simulink library "tether005_ul"  (R2020a)
settings: Solver=VariableStepAuto  StartTime=0.0  StopTime=10.0  RelTol=1e-3
values from neighbouring files (symbols this model uses):
  initNodePos = [INITIALLINE;INITIALLINE;INITIALLINE]    [tether005_ts.m]
  initNodeVel = [zeros(1,numNodes-2);zeros(1,numNodes-2);zeros(1,numNodes-2)]    [tether005_ts.m]
  numNodes = 11    [tether005_ts.m]
libraries: powerlib_meascontrol x2
settings Model: Creator=mitch  LastModifiedBy=mr-jo

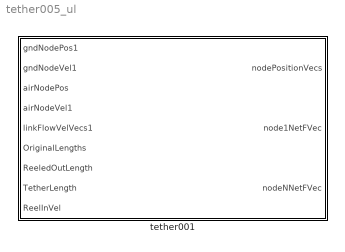
== system tether005_ul ==
  tether001 : Subsystem

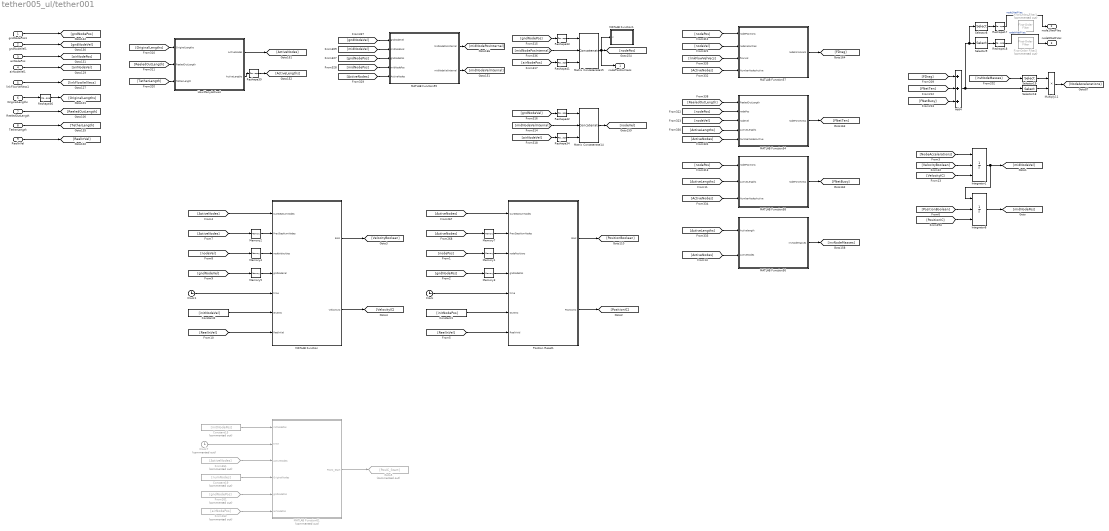
== system tether005_ul/tether001 ==
  gndNodePos1 : Inport
  gndNodeVel1 : Inport  Port=2
  airNodePos : Inport  Port=3
  airNodeVel1 : Inport  Port=4
  linkFlowVelVecs1 : Inport  Port=5
  OriginalLengths : Inport  Port=6
  ReeledOutLength : Inport  Port=7
  TetherLength : Inport  Port=8
  ReelInVel : Inport  Port=9
  Add4 : Sum  Inputs=3
  Clock : Clock
  Clock1 : Clock
  Clock7 : Clock  Commented=on
  Constant1 : Constant  Value=[initNodePos]
  Constant15 : Constant  Commented=on  Value=[initNodePos]
  Constant19 : Constant  Commented=on  Value=[numNodes]
  Constant2 : Constant  Value=[initNodeVel]
  First-Order Filter1 : powerlib_meascontrol/Filters/First-Order Filter  Commented=on  FilterType=Lowpass  Tc=1  Ts=0  Initialize=on  Vac_Init=[0, 0, 60]  Vdc_Init=0  PlotResponse=off  FreqRange="[0,  200,  1]"
  First-Order Filter2 : powerlib_meascontrol/Filters/First-Order Filter  Commented=on  FilterType=Lowpass  Tc=1  Ts=0  Initialize=on  Vac_Init=[0, 0, 60]  Vdc_Init=0  PlotResponse=off  FreqRange="[0,  200,  1]"
  From161 : From  Commented=on  GotoTag=gndNodePos
  From162 : From  Commented=on  GotoTag=airNodePos
  From361 : From  Commented=on  GotoTag=ActiveNodes
  Goto5 : Goto  Commented=on  GotoTag=PosIC_Start
  HowManyActive4 : MATLAB Function  TreatAsAtomicUnit=on
  Integrator1 : Integrator  ExternalReset=rising  InitialConditionSource=external
  Integrator8 : Integrator  ExternalReset=rising  InitialConditionSource=external
  MATLAB Function : MATLAB Function  TreatAsAtomicUnit=on
  MATLAB Function1 : MATLAB Function  TreatAsAtomicUnit=on
  MATLAB Function54 : MATLAB Function  TreatAsAtomicUnit=on
  MATLAB Function55 : MATLAB Function  TreatAsAtomicUnit=on
  MATLAB Function56 : MATLAB Function  TreatAsAtomicUnit=on
  MATLAB Function57 : MATLAB Function  TreatAsAtomicUnit=on
  MATLAB Function58 : MATLAB Function  TreatAsAtomicUnit=on
  MATLAB Function61 : MATLAB Function  Commented=on  TreatAsAtomicUnit=on
  Matrix Concatenate14 : Concatenate  NumInputs=3  Mode=Multidimensional array  ConcatenateDimension=2
  Matrix Concatenate15 : Concatenate  NumInputs=3  Mode=Multidimensional array  ConcatenateDimension=2
  Memory{1..5,7} (6 alike) : Memory
  Multiply11 : Product
  Position Reset1 : MATLAB Function  TreatAsAtomicUnit=on
  Reshape{17..18,33..34,41..42} (6 alike) : Reshape  OutputDimensionality=Column vector (2-D)
  Reshape36 : Reshape  OutputDimensionality=Row vector (2-D)
  Reshape39 : Reshape  OutputDimensionality=Row vector (2-D)
  Selector18 : Selector  NumberOfDimensions=2  InputPortWidth=3  IndexOptions=Select all,Index vector (dialog)  Indices=[1 3],2:numNodes-1  OutputSizes=1,1
  Selector19 : Selector  NumberOfDimensions=2  InputPortWidth=3  IndexOptions=Select all,Index vector (dialog)  Indices=[1 3],2:numNodes-1  OutputSizes=1,1
  Selector8 : Selector  NumberOfDimensions=2  InputPortWidth=3  IndexOptions=Select all,Index vector (dialog)  Indices=[1 3],1  OutputSizes=1,1
  Selector9 : Selector  NumberOfDimensions=2  InputPortWidth=3  IndexOptions=Select all,Starting index (dialog)  Indices=[1 3],numNodes  OutputSizes=1,1
  nodePositionVecs : Outport  VectorParamsAs1DForOutWhenUnconnected=off
  node1NetFVec : Outport  Port=2  VectorParamsAs1DForOutWhenUnconnected=off
  nodeNNetFVec : Outport  Port=3  VectorParamsAs1DForOutWhenUnconnected=off
  wires:
  ? -> ?
  [gndNodeVel] -> Reshape42/1
  [ActiveNodes] -> MATLAB Function54/5(NumberNodesActive)
  MATLAB Function56/1(invNodeMasses) -> [invNodeMasses]
  [gndNodePos] -> Reshape33/1
  HowManyActive4/2(ActiveLengths) -> Reshape39/1
  [airNodePos] -> Reshape41/1
  [midNodePosInternal] -> Matrix Concatenate15/2
  [nodePos] -> MATLAB Function57/1(nodePositions)
  [ActiveLengths] -> MATLAB Function56/1(Activelength)
  MATLAB Function58/1(nodeForceVecs) -> [FNetBuoy]
  [ReeledOutLength] -> HowManyActive4/2(ReeledOutLength)
  Reshape42/1 -> Matrix Concatenate14/1
  [ActiveNodes] -> MATLAB Function58/3(NumberNodesActive)
  Reshape39/1 -> [ActiveLengths]
  Reshape41/1 -> Matrix Concatenate15/3
  Reshape33/1 -> Matrix Concatenate15/1
  [airNodeVel] -> Reshape34/1
  [nodeVel] -> MATLAB Function54/3(nodeVel)
  Matrix Concatenate14/1 -> [nodeVel]
  MATLAB Function54/1(nodeForceVecs) -> [FNetTen]
  [nodePos] -> MATLAB Function58/1(nodePositions)
  Matrix Concatenate15/1 -> MATLAB Function1/1(u), [nodePos], nodePositionVecs/1
  [ActiveLengths] -> MATLAB Function54/4(ActiveLengths)
  [gndNodeVel] -> MATLAB Function55/1(gndNodeVel)
  HowManyActive4/1(ActiveNodes) -> [ActiveNodes]
  [midNodePos] -> MATLAB Function55/4(midNodePos)
  [ActiveNodes] -> MATLAB Function55/5(ActiveNodes)
  [midNodeVelInternal] -> Matrix Concatenate14/2
  [gndNodePos] -> MATLAB Function55/3(gndNodePos)
  Reshape34/1 -> Matrix Concatenate14/3
  [nodeVel] -> MATLAB Function57/2(nodeVelocities)
  [TetherLength] -> HowManyActive4/3(TetherLength)
  [ActiveNodes] -> MATLAB Function57/4(NumberNodesActive)
  [ReeledOutLength] -> MATLAB Function54/1(ReeledOutLength)
  MATLAB Function55/2(midNodeVelInternal) -> [midNodeVelInternal]
  [nodePos] -> MATLAB Function54/2(nodePos)
  [midNodeVel] -> MATLAB Function55/2(midNodeVel)
  MATLAB Function57/1(nodeForceVecs) -> [FDrag]
  [linkFlowVelVecs] -> MATLAB Function57/3(flowVel)
  [OriginalLengths] -> HowManyActive4/1(OriginalLengths)
  ReeledOutLength/1 -> [ReeledOutLength]
  Reshape36/1 -> [OriginalLengths]
  gndNodePos1/1 -> [gndNodePos]
  gndNodeVel1/1 -> [gndNodeVel]
  airNodePos/1 -> [airNodePos]
  airNodeVel1/1 -> [airNodeVel]
  linkFlowVelVecs1/1 -> [linkFlowVelVecs]
  OriginalLengths/1 -> Reshape36/1
  TetherLength/1 -> [TetherLength]
  ReelInVel/1 -> [ReelInVel]
  MATLAB Function55/1(midNodePosInternal) -> [midNodePosInternal]
  [ActiveNodes] -> Position Reset1/1(CurStepNumNodes)
  Position Reset1/1(Bool) -> [PositionBoolean]
  [ActiveNodes] -> Memory7/1
  Selector18/1 -> Multiply11/2
  Memory7/1 -> Position Reset1/2(PrevStepNumNodes)
  [invNodeMasses] -> Selector19/1
  Selector19/1 -> Multiply11/1
  [FNetTen] -> Add4/2
  Add4/1 -> Selector9/1, Selector8/1, Selector18/1
  [FDrag] -> Add4/1
  Multiply11/1 -> [NodeAccelerations]
  [FNetBuoy] -> Add4/3
  [NodeAccelerations] -> Integrator1/1
  Integrator8/1 -> [midNodePos]
  [gndNodePos] -> Memory3/1
  Position Reset1/2(PositionIC) -> [PositionIC]
  Clock/1 -> Position Reset1/5(time)
  [PositionIC] -> Integrator8/3
  Memory3/1 -> Position Reset1/4(gndNodePos)
  [ReelInVel] -> Position Reset1/7(ReelInVel)
  Selector8/1 -> Reshape17/1
  Selector9/1 -> Reshape18/1
  Integrator1/1 -> Integrator8/1, [midNodeVel]
  [PositionBoolean] -> Integrator8/2
  [ActiveNodes] -> MATLAB Function/1(CurStepNumNodes)
  [ActiveNodes] -> Memory2/1
  Memory2/1 -> MATLAB Function/2(PrevStepNumNodes)
  [nodeVel] -> Memory4/1
  Memory4/1 -> MATLAB Function/3(nodeVelocities)
  [gndNodeVel] -> Memory5/1
  Memory5/1 -> MATLAB Function/4(gndNodeVel)
  Clock1/1 -> MATLAB Function/5(time)
  Constant2/1 -> MATLAB Function/6(GivenIC)
  [ReelInVel] -> MATLAB Function/7(ReelInVel)
  MATLAB Function/1(Bool) -> [VelocityBoolean]
  MATLAB Function/2(VelocityIC) -> [VelocityIC]
  [VelocityIC] -> Integrator1/3
  [VelocityBoolean] -> Integrator1/2
  [ActiveLengths] -> MATLAB Function58/2(ActiveLengths)
  [ActiveNodes] -> MATLAB Function56/2(ActiveNodes)
  [nodePos] -> Memory1/1
  Memory1/1 -> Position Reset1/3(nodePositions)
  From361/1 -> MATLAB Function61/3(ActiveNodes)
  Constant19/1 -> MATLAB Function61/4(OriginalNodes)
  From162/1 -> MATLAB Function61/6(airNodePos)
  Clock7/1 -> MATLAB Function61/2(time)
  From161/1 -> MATLAB Function61/5(gndNodePos)
  Constant15/1 -> MATLAB Function61/1(initNodePos)
  MATLAB Function61/1(PosIC_Start) -> Goto5/1
  Constant1/1 -> Position Reset1/6(GivenIC)
  Reshape18/1 -> nodeNNetFVec/1  "nodeNNetFVec"
  Reshape17/1 -> node1NetFVec/1  "node1NetFVec"

== matlab function tether005_ul/tether001/MATLAB Function1 ==
  data: u input
function  fcn(u)

u;

== matlab function tether005_ul/tether001/MATLAB Function61 ==
  data: initNodePos input size=[3,numNodes-2]; time input size=1; ActiveNodes input size=1; OriginalNodes input size=1; gndNodePos input size=[3,1]; airNodePos input size=[3,1]; PosIC_Start output
function PosIC_Start = fcn(initNodePos,time, ActiveNodes, OriginalNodes,gndNodePos,airNodePos)

if time==0
    Na = ActiveNodes;
    No = 11;%OriginalNodes;
    
    TetherVec = [linspace(gndNodePos(1),airNodePos(1),Na);...
                 linspace(gndNodePos(2),airNodePos(2),Na);...
                 linspace(gndNodePos(3),airNodePos(3),Na)];
    PosIC_Start = [gndNodePos(1)*ones(1,No-2);...
             gndNodePos(2)*ones(1,No-2);...
             gndNodePos(3)*ones(1,No-2)];

    % initNodePos   
    PosIC_Start(1,((No-Na)+1):end) = linspace(TetherVec(1,2),TetherVec(1,end-1),Na-2);
    PosIC_Start(2,((No-Na)+1):end) = linspace(TetherVec(2,2),TetherVec(2,end-1),Na-2);
    PosIC_Start(3,((No-Na)+1):end) = linspace(TetherVec(3,2),TetherVec(3,end-1),Na-2);
else
    PosIC_Start = zeros(3,size(initNodePos,2));
end

== matlab function tether005_ul/tether001/Position Reset1 ==
  data: CurStepNumNodes input; Bool output; PrevStepNumNodes input; nodePositions input; gndNodePos input; PositionIC output; time input; GivenIC input; ReelInVel input
function [Bool,PositionIC]  = fcn(CurStepNumNodes, PrevStepNumNodes, nodePositions, gndNodePos, time, GivenIC, ReelInVel)

if ReelInVel<=0
    if time==0
        PositionIC = GivenIC;
        Bool = 1;
    else
        Na = CurStepNumNodes;
        No = size(nodePositions,2);

        if PrevStepNumNodes==0
            Nc = CurStepNumNodes;
            Np = Nc;
        else
            Np = PrevStepNumNodes;
            Nc = CurStepNumNodes;
        end

        PositionIC = [gndNodePos(1)*ones(1,No-2);...
                      gndNodePos(2)*ones(1,No-2);...
                      gndNodePos(3)*ones(1,No-2)];

        % Checks If The Current Number of Nodes Equals Previous Number of Nodes
        % If not equal then reset initial conditions
        if Nc == Np
            Bool = -1;
        else
            Bool = 1;
            linkVecs  = diff(nodePositions,1,2);
            for ii = 1:(Na-2)
                jj = (Na-2)-ii+1;
                VecToi = sum(linkVecs(:,1:(No-ii-2)),2);
                VecNextPercent = linkVecs(:,No-ii-1).*(jj/(Na-1));
                PositionIC(:,jj+(No-Na)) = VecToi+VecNextPercent;              
            end  
        end
    end         
else
    if time==0
        PositionIC = GivenIC;
        Bool = 1;
    else
        Na = CurStepNumNodes;
        No = size(nodePositions,2);

        if PrevStepNumNodes==0
            Nc = CurStepNumNodes;
            Np = Nc;
        else
            Np = PrevStepNumNodes;
            Nc = CurStepNumNodes;
        end

        PositionIC = [gndNodePos(1)*ones(1,No-2);...
                      gndNodePos(2)*ones(1,No-2);...
                      gndNodePos(3)*ones(1,No-2)];
                  
        % Checks If The Current Number of Nodes Equals Previous Number of Nodes
        % If not equal then reset initial conditions
        if Nc == Np
            Bool = -1;
        else
            Bool = 1;
            linkVecs  = diff(nodePositions,1,2);
            for ii = 1:(Na-2)
                jj = (Na-2)-ii+1;
                VecToi = sum(linkVecs(:,1:(No-ii)),2);
                VecNextPercent = linkVecs(:,No-ii).*((jj)/(Na-1));
                PositionIC(:,jj+(No-Na)) = VecToi-VecNextPercent;
            end 
        end
    end  
end
%%%%%%%%%%%%%%%%%%%%%%%%


if Bool == 1
    diff(PositionIC,1,2);
end

== matlab function tether005_ul/tether001/HowManyActive4 ==
  data: OriginalLengths input; ActiveNodes output; ReeledOutLength input; ActiveLengths output; TetherLength input
function [ActiveNodes, ActiveLengths] = fcn(OriginalLengths, ReeledOutLength, TetherLength)

OriginalNodes = length(OriginalLengths)+1;
No = OriginalNodes;

ActiveLengths = zeros(size(OriginalLengths));
L = zeros(size(ActiveLengths));
flag = false;
a = 1;

if ReeledOutLength == TetherLength
    a = a+1;
    L(1:end) = OriginalLengths(1:end);
else
    while flag == false
        if ReeledOutLength == sum(OriginalLengths(a:end))
            flag = true;
        elseif ReeledOutLength > sum(OriginalLengths(a:end))
            flag = true;
        else
            a=a+1;
        end
    end

L((a-1):end) = (ReeledOutLength/(No-a+1))*ones(1,(No-a+1));

end

ActiveNodes = nnz(L)+1;
ActiveLengths = L;

== matlab function tether005_ul/tether001/MATLAB Function54 ==
  data: ReeledOutLength input; nodePos input; nodeForceVecs output; nodeVel input; ActiveLengths input; NumberNodesActive input
function nodeForceVecs  = fcn(ReeledOutLength, nodePos, nodeVel, ActiveLengths, NumberNodesActive)

mass = .05;
zeta = .75;
diameter = .0144;
youngsMod = 5*10^10;

TotalNodes = size(nodePos,2);
No = TotalNodes;
Na = NumberNodesActive;

unstretchedLength = ReeledOutLength;
totalSpringConst = youngsMod*(pi/4)*(diameter^2)/unstretchedLength;

SpringConsts = zeros(1,TotalNodes-1);
if Na>2
    SpringConsts(:,(No-Na+1):end) = youngsMod*(pi/4)*(diameter^2)./ActiveLengths(1,(end-NumberNodesActive+2):end);
else
    SpringConsts(end) = totalSpringConst;
end
DampCoeffs = zeta*2*sqrt(SpringConsts.*mass);

linkVecs  = diff(nodePos,1,2);
linkLength = sqrt(sum(linkVecs.^2));

linkUnitVecs = zeros(3,TotalNodes-1);
linkUnitVecs(1:3,(No-Na+1):end) = linkVecs(1:3,(No-Na+1):end)./repmat(sqrt(sum((linkVecs(1:3,(No-Na+1):end).^2),1)),[3 1]);
%prevent divide by zero if reeled in 
linkUnitVecs(isnan(linkUnitVecs))=0;

%Rate of change of all links
linkLengthDeriv = dot(nodeVel(:,2:end)-nodeVel(:,1:end-1),linkUnitVecs);

%Forces from spring and damping in each link
springForces = SpringConsts.*(linkLength-ActiveLengths);
damperForces = DampCoeffs.*linkLengthDeriv;

%Finds force along each link
totalLinkForceVec = repmat(springForces+damperForces,[3 1]).*linkUnitVecs;

%Finds force on each node
nodeForceVecs = [totalLinkForceVec(:,1) diff(totalLinkForceVec,1,2) -totalLinkForceVec(:,end)];

%Moves Reeled in bottom  node force to Ground Node
if SpringConsts(1) == 0
    nodeForceVecs(:,1) = nodeForceVecs(:,No-Na+1);
    nodeForceVecs(:,No-Na+1) = [0;0;0];
end

== matlab function tether005_ul/tether001/MATLAB Function55 ==
  data: gndNodeVel input size=[3,1]; midNodeVel input size=[3,numNodes-2]; gndNodePos input size=[3,1]; midNodePosInternal output size=[3,numNodes-2]; midNodePos input size=[3,numNodes-2]; ActiveNodes input size=1; midNodeVelInternal output size=[3,numNodes-2]
function [midNodePosInternal,  midNodeVelInternal] = fcn(gndNodeVel,midNodeVel,gndNodePos, midNodePos, ActiveNodes)

No = size(midNodePos,2)+2;
Na = ActiveNodes;

% Reeled In Nodes are ground
midNodePosInternal = [gndNodePos(1)*ones(1,No-2);...
                      gndNodePos(2)*ones(1,No-2);...
                      gndNodePos(3)*ones(1,No-2)];
                  
midNodeVelInternal = [gndNodeVel(1)*ones(1,No-2);...
                      gndNodeVel(2)*ones(1,No-2);...
                      gndNodeVel(3)*ones(1,No-2)];              
                  
% Given for unalternd nodes
midNodePosInternal(:,((No-Na)+1):end) = midNodePos(:,((No-Na)+1):end);
midNodeVelInternal(:,((No-Na)+1):end) = midNodeVel(:,((No-Na)+1):end);

== matlab function tether005_ul/tether001/MATLAB Function56 ==
  data: invNodeMasses output; Activelength input; ActiveNodes input
function invNodeMasses  = fcn(Activelength,ActiveNodes)

tetherDensity = 952;
diameter = .0144;

Na = ActiveNodes;
No = length(Activelength)+1;

% Mass of each link, 1xN-1
linkMasses  = tetherDensity*(Activelength*(pi/4)*diameter^2);

% 1/mass for each node, 3xN (repmat so that we can multiply with force
% vectors concatenated into matrix later
invNodeMasses = zeros(3,No);
invNodeMasses(:,(No-Na+1):end) = repmat(1./([linkMasses((No-Na+1)) linkMasses((No-Na+1):end-1)+linkMasses((No-Na+2):end) linkMasses(end)]/2),[3 1]);

%Make Zero Inverse mass also equal to zero
for i = 1:size(invNodeMasses,2)
    if invNodeMasses(:,i) == Inf
        invNodeMasses(:,i) = zeros(3,1);
    end
end

%makes bottom node mass on ground node
if invNodeMasses(:,1) == 0
    invNodeMasses(:,1) = invNodeMasses(:,No-Na+1);
    invNodeMasses(:,No-Na+1) = [0;0;0];
end

== matlab function tether005_ul/tether001/MATLAB Function57 ==
  data: nodePositions input size=[3,numNodes]; nodeVelocities input size=[3,numNodes]; flowVel input; NumberNodesActive input; nodeForceVecs output
function nodeForceVecs = fcn(nodePositions,nodeVelocities, flowVel, NumberNodesActive)

flowDensity = 1025;
dragCoeff = .5;
thrDiam = .0144;

TotalNodes = size(nodePositions,2);
No = TotalNodes;
Na = NumberNodesActive;

% Velocity and center of links 3xN-1
linkVelocities = (nodeVelocities(:,1:end-1) + nodeVelocities(:,2:end))/2;

% Apparent flow at center of links 3xN-1
linkAppFlow = flowVel - linkVelocities; 

% Link center apparent flow magnitude 3xN-1
linkAppFlowMag = sqrt(sum(linkAppFlow.^2)); % Sum over columns

% Normalize columns to get unit vector 3xN-1
dragDirUnitVec = linkAppFlow./repmat(linkAppFlowMag,[3 1]);
dragDirUnitVec(isnan(dragDirUnitVec)) = 0;

% Dynamic pressures at link centers 1xN-1
dynPress = 0.5*flowDensity*linkAppFlowMag.^2;

%Vector Between All Nodes
linkVecs  = diff(nodePositions,1,2);

% Link lengths, diff over columns 1xN-1
linkLengths = sqrt(sum(diff(nodePositions,1,2).^2));

% Unit vectors in the direction of the link 3xN-1
linkUnitVecs = zeros(3,TotalNodes-1);
linkUnitVecs(1:3,(end-NumberNodesActive+2):end) = linkVecs(1:3,(end-NumberNodesActive+2):end)./repmat(sqrt(sum((linkVecs(1:3,(end-NumberNodesActive+2):end).^2),1)),[3 1]);

%Check for reeled in Nodes prevent divide by zero
linkUnitVecs(isnan(linkUnitVecs))=0;

% Projected areas of each link
projArea = thrDiam*linkLengths.*sqrt(sum(cross(linkUnitVecs,dragDirUnitVec).^2,1));

% Drag force on links
linkForceVecs = repmat(dragCoeff*dynPress.*projArea,[3 1]).*dragDirUnitVec;

% Drag force on nodes
nodeForceVecs = zeros(3,TotalNodes);
nodeForceVecs(:,(TotalNodes-NumberNodesActive+1):end) = [linkForceVecs(:,(TotalNodes-NumberNodesActive+1)), (linkForceVecs(:,((TotalNodes-NumberNodesActive+1)):end-1)+linkForceVecs(:,((TotalNodes-NumberNodesActive+2)):end)) linkForceVecs(:,end)]/2;

%Moves Reeled in bottom Node to Ground Node
if NumberNodesActive<TotalNodes
    nodeForceVecs(:,1) = nodeForceVecs(:,No-Na+1);
    nodeForceVecs(:,No-Na+1) = [0;0;0];
end

== matlab function tether005_ul/tether001/MATLAB Function58 ==
  data: nodePositions input; ActiveLengths input; NumberNodesActive input; nodeForceVecs output
function nodeForceVecs = fcn(nodePositions,ActiveLengths, NumberNodesActive)

tetherDensity = 952;
fluidDensity = 1025;
diameter = .0144;
gravity = 9.81;

% In this notation, N is the number of nodes
Na = NumberNodesActive;
No = size(nodePositions,2);

% Actual Length of each link 1xN-1
linkLengths = sqrt(sum(diff(nodePositions,1,2).^2));

% Number of links, scalar
numLinks = size(linkLengths,2);

% Volume of each link, 1xN-1
Volumes  = ActiveLengths.*(pi/4)*diameter^2;

% Mass of each link, 1xN-1
linkMasses = tetherDensity*Volumes;

% Net force on the links (Buoyancy - Weight) on each link, 3xN-1
linkNetForceVecs = [repmat([0 0]',[1 numLinks]);(-gravity*linkMasses + gravity*fluidDensity*Volumes)];

% Net force on the nodes, 3xN
nodeForceVecs = [linkNetForceVecs(:,1) linkNetForceVecs(:,1:end-1)+linkNetForceVecs(:,2:end) linkNetForceVecs(:,end)]/2;

% Moves bottome node force to ground force
if linkMasses(1) == 0
    nodeForceVecs(:,1) = nodeForceVecs(:,No-Na+1);
    nodeForceVecs(:,No-Na+1) = [0;0;0];
end

== matlab function tether005_ul/tether001/MATLAB Function ==
  data: CurStepNumNodes input; Bool output; PrevStepNumNodes input; nodeVelocities input; gndNodeVel input; time input; GivenIC input; ReelInVel input; VelocityIC output
function [Bool,VelocityIC]  = fcn(CurStepNumNodes, PrevStepNumNodes, nodeVelocities, gndNodeVel, time, GivenIC, ReelInVel)

if ReelInVel<=0
    if time==0
        VelocityIC = GivenIC;
        Bool = 1;
    else
        Na = CurStepNumNodes;
        No = size(nodeVelocities,2);

        if PrevStepNumNodes==0
            Nc = CurStepNumNodes;
            Np = Nc;
        else
            Np = PrevStepNumNodes;
            Nc = CurStepNumNodes;
        end

        VelocityIC = [gndNodeVel(1)*ones(1,No-2);...
                      gndNodeVel(2)*ones(1,No-2);...
                      gndNodeVel(3)*ones(1,No-2)];

        % Checks If The Current Number of Nodes Equals Previous Number of Nodes
        % If not equal then reset initial conditions
        if Nc == Np
            Bool = -1;
        else
            Bool = 1;
            linkVecs  = diff(nodeVelocities,1,2);
            for ii = 1:(Na-2)
                jj = (Na-2)-ii+1;
                VecToi = sum(linkVecs(:,1:(No-ii-2)),2);
                VecNextPercent = linkVecs(:,No-ii-1).*(jj/(Na-1));
                VelocityIC(:,jj+(No-Na)) = VecToi+VecNextPercent;
            end  
        end
    end         
else
    if time==0
        VelocityIC = GivenIC;
        Bool = 1;
    else
        Na = CurStepNumNodes;
        No = size(nodeVelocities,2);

        if PrevStepNumNodes==0
            Nc = CurStepNumNodes;
            Np = Nc;
        else
            Np = PrevStepNumNodes;
            Nc = CurStepNumNodes;
        end

        VelocityIC = [gndNodeVel(1)*ones(1,No-2);...
                      gndNodeVel(2)*ones(1,No-2);...
                      gndNodeVel(3)*ones(1,No-2)];
                  
        % Checks If The Current Number of Nodes Equals Previous Number of Nodes
        % If not equal then reset initial conditions
        if Nc == Np
            Bool = -1;
        else
            Bool = 1;
            linkVecs  = diff(nodeVelocities,1,2);
            for ii = 1:(Na-2)
                jj = (Na-2)-ii+1;
                VecToi = sum(linkVecs(:,1:(No-ii)),2);
                VecNextPercent = linkVecs(:,No-ii).*((jj)/(Na-1));
                VelocityIC(:,jj+(No-Na)) = VecToi-VecNextPercent;
            end 
        end
    end  
end
